simulink model "DatcomNew"  (R2017a)
settings: Solver=VariableStepAuto  StartTime=0.0  StopTime=10.0  RelTol=1e-3
undefined symbols (not defined in the file or in its folder): datcom, Newton, Raphson
libraries: aerolibutil x32, sharedutil x4, aerolibtransform2 x3, aerolibasang x3, aerolibadyn x1
(part 1 of 4)
settings Model: Creator=AHKh  LastModifiedBy=AHKh

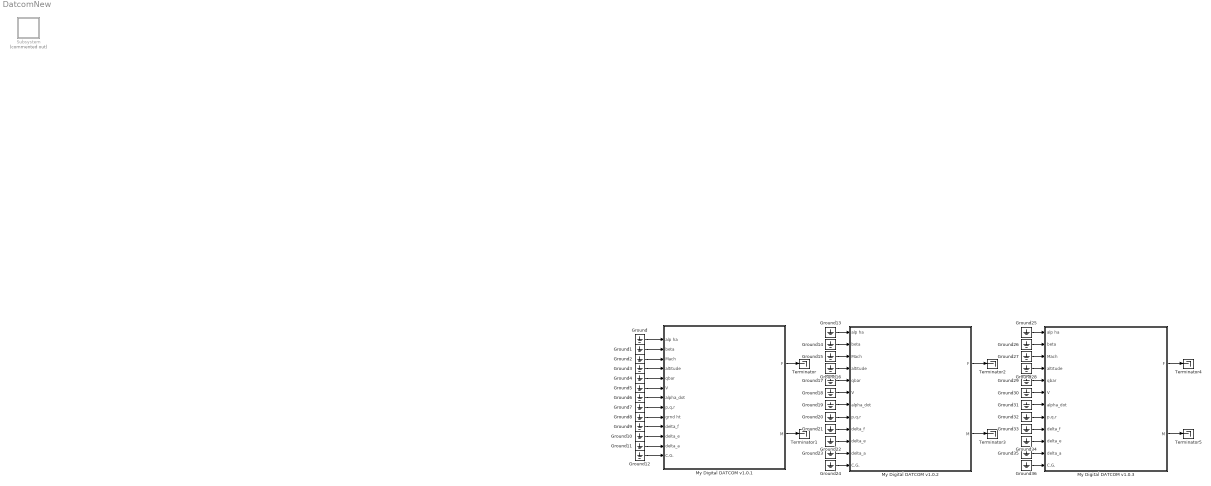
== system DatcomNew ==
  Ground{,1..36} (37 alike) : Ground
  My Digital DATCOM v1.0.1 : Subsystem  mask{datcom=datcom}
      mask prompts: datcom "Datcom Structure"
      mask Display:
      | port_label('input',1,'\alpha (rad)','texmode','on');
      | port_label('input',2,'\beta (rad)','texmode','on');
      | port_label('input',3,'Mach','texmode','on');
      | port_label('input',4,'h (m)','texmode','on');
      | port_label('input',5,'q_{bar}','texmode','on');
      | port_label('input',6,'V_{body} m/s','texmode','on');
      | port_label('input',7,'d\alpha/dt (rad/s)','texmode','on');
      | port_label('input',8,'\omega (rad/s)','texmode','on');
      | port_label('input',9,'h_{grnd} (m)','texmode','on');
      | port_label('input',10,'\delta_F (rad)','texmode','on');
      | port_label('input',11,'\delta_E (rad)','texmode','on');
      | port_label('input',12,'\delta_A (rad)','texmode','on');
      | port_label('input',13,'C.G. (m)','texmode','on');
      | port_label('output',1,'F_{body} (N)','texmode','on');
      | port_label('output',2,'M_{body} (N.m)','texmode','on');
  My Digital DATCOM v1.0.2 : Subsystem  mask{datcom=datcom}
      mask prompts: datcom "Datcom Structure"
      mask Display:
      | port_label('input',1,'\alpha (rad)','texmode','on');
      | port_label('input',2,'\beta (rad)','texmode','on');
      | port_label('input',3,'Mach','texmode','on');
      | port_label('input',4,'h (m)','texmode','on');
      | port_label('input',5,'q_{bar}','texmode','on');
      | port_label('input',6,'V_{body} m/s','texmode','on');
      | port_label('input',7,'d\alpha/dt (rad/s)','texmode','on');
      | port_label('input',8,'\omega (rad/s)','texmode','on');
      | port_label('input',9,'\delta_F (rad)','texmode','on');
      | port_label('input',10,'\delta_E (rad)','texmode','on');
      | port_label('input',11,'\delta_A (rad)','texmode','on');
      | port_label('input',12,'C.G. (m)','texmode','on');
      | port_label('output',1,'F_{body} (N)','texmode','on');
      | port_label('output',2,'M_{body} (N.m)','texmode','on');
  My Digital DATCOM v1.0.3 : Subsystem  mask{datcom=datcom}
      mask prompts: datcom "Datcom Structure"
      mask Display:
      | port_label('input',1,'\alpha (rad)','texmode','on');
      | port_label('input',2,'\beta (rad)','texmode','on');
      | port_label('input',3,'Mach','texmode','on');
      | port_label('input',4,'h (m)','texmode','on');
      | port_label('input',5,'q_{bar}','texmode','on');
      | port_label('input',6,'V_{body} m/s','texmode','on');
      | port_label('input',7,'d\alpha/dt (rad/s)','texmode','on');
      | port_label('input',8,'\omega (rad/s)','texmode','on');
      | port_label('input',9,'\delta_F (rad)','texmode','on');
      | port_label('input',10,'\delta_E (rad)','texmode','on');
      | port_label('input',11,'\delta_A (rad)','texmode','on');
      | port_label('input',12,'C.G. (m)','texmode','on');
      | port_label('output',1,'F_{body} (N)','texmode','on');
      | port_label('output',2,'M_{body} (N.m)','texmode','on');
  Subsystem : Subsystem  Commented=on
  Terminator{,1..5} (6 alike) : Terminator
  wires:
  My Digital DATCOM v1.0.1/2(M) -> Terminator1/1
  My Digital DATCOM v1.0.1/1(F) -> Terminator/1
  Ground4/1 -> My Digital DATCOM v1.0.1/5(qbar)
  Ground5/1 -> My Digital DATCOM v1.0.1/6(V)
  Ground/1 -> My Digital DATCOM v1.0.1/1(alp ha)
  Ground3/1 -> My Digital DATCOM v1.0.1/4(altitude)
  Ground7/1 -> My Digital DATCOM v1.0.1/8(p,q,r)
  Ground12/1 -> My Digital DATCOM v1.0.1/13(C.G.)
  Ground8/1 -> My Digital DATCOM v1.0.1/9(grnd ht)
  Ground6/1 -> My Digital DATCOM v1.0.1/7(alpha_dot)
  Ground1/1 -> My Digital DATCOM v1.0.1/2(beta)
  Ground2/1 -> My Digital DATCOM v1.0.1/3(Mach)
  Ground9/1 -> My Digital DATCOM v1.0.1/10(delta_f)
  Ground10/1 -> My Digital DATCOM v1.0.1/11(delta_e)
  Ground11/1 -> My Digital DATCOM v1.0.1/12(delta_a)
  My Digital DATCOM v1.0.2/1(F) -> Terminator2/1
  My Digital DATCOM v1.0.2/2(M) -> Terminator3/1
  Ground13/1 -> My Digital DATCOM v1.0.2/1(alp ha)
  Ground16/1 -> My Digital DATCOM v1.0.2/4(altitude)
  Ground19/1 -> My Digital DATCOM v1.0.2/7(alpha_dot)
  Ground18/1 -> My Digital DATCOM v1.0.2/6(V)
  Ground14/1 -> My Digital DATCOM v1.0.2/2(beta)
  Ground15/1 -> My Digital DATCOM v1.0.2/3(Mach)
  Ground17/1 -> My Digital DATCOM v1.0.2/5(qbar)
  Ground20/1 -> My Digital DATCOM v1.0.2/8(p,q,r)
  Ground22/1 -> My Digital DATCOM v1.0.2/10(delta_e)
  Ground21/1 -> My Digital DATCOM v1.0.2/9(delta_f)
  Ground24/1 -> My Digital DATCOM v1.0.2/12(C.G.)
  Ground23/1 -> My Digital DATCOM v1.0.2/11(delta_a)
  Ground27/1 -> My Digital DATCOM v1.0.3/3(Mach)
  My Digital DATCOM v1.0.3/2(M) -> Terminator5/1
  My Digital DATCOM v1.0.3/1(F) -> Terminator4/1
  Ground32/1 -> My Digital DATCOM v1.0.3/8(p,q,r)
  Ground26/1 -> My Digital DATCOM v1.0.3/2(beta)
  Ground33/1 -> My Digital DATCOM v1.0.3/9(delta_f)
  Ground29/1 -> My Digital DATCOM v1.0.3/5(qbar)
  Ground35/1 -> My Digital DATCOM v1.0.3/11(delta_a)
  Ground25/1 -> My Digital DATCOM v1.0.3/1(alp ha)
  Ground36/1 -> My Digital DATCOM v1.0.3/12(C.G.)
  Ground31/1 -> My Digital DATCOM v1.0.3/7(alpha_dot)
  Ground30/1 -> My Digital DATCOM v1.0.3/6(V)
  Ground28/1 -> My Digital DATCOM v1.0.3/4(altitude)
  Ground34/1 -> My Digital DATCOM v1.0.3/10(delta_e)

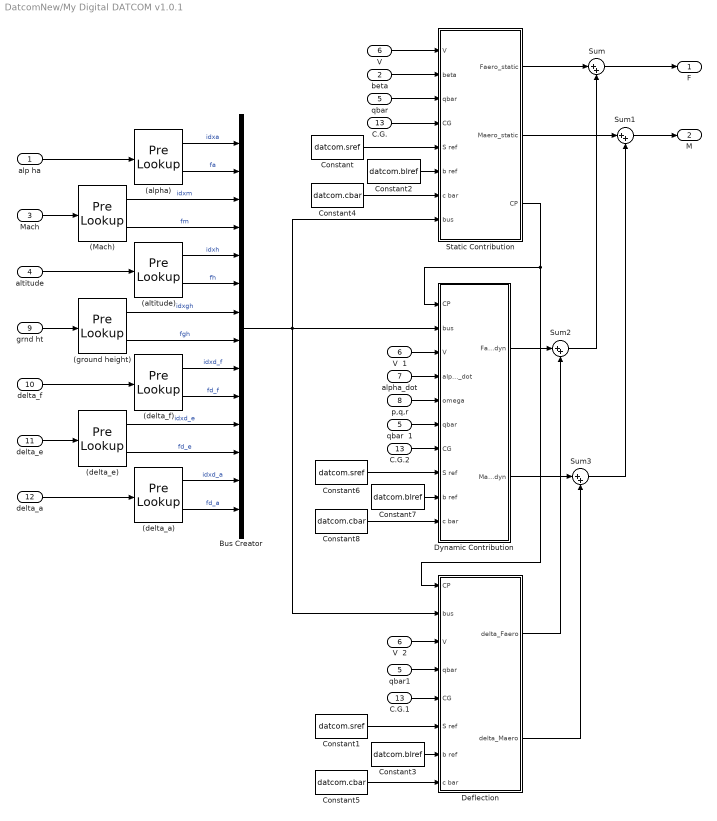
== system DatcomNew/My Digital DATCOM v1.0.1 ==
  alp ha : Inport  Unit=rad
  beta : Inport  Port=2  Unit=rad
  Mach : Inport  Port=3  Unit=1
  altitude : Inport  Port=4  Unit=m
  qbar : Inport  Port=5  Unit=Pa
  V : Inport  Port=6  Unit=m/s
  alpha_dot : Inport  Port=7  Unit=rad/s
  p,q,r : Inport  Port=8  Unit=rad/s
  grnd ht : Inport  Port=9  Unit=m
  delta_f : Inport  Port=10  Unit=rad
  delta_e : Inport  Port=11  Unit=rad
  delta_a : Inport  Port=12  Unit=rad
  C.G. : Inport  Port=13  Unit=m
  (Mach) : PreLookup  BreakpointsData=datcom.mach  BeginIndexSearchUsingPreviousIndexResult=on  IndexDataTypeStr=int32  FractionDataTypeStr=double
  (alpha) : PreLookup  BreakpointsData=datcom.alpha  BeginIndexSearchUsingPreviousIndexResult=on  IndexDataTypeStr=int32  FractionDataTypeStr=double
  (altitude) : PreLookup  BreakpointsData=datcom.alt  BeginIndexSearchUsingPreviousIndexResult=on  IndexDataTypeStr=int32  FractionDataTypeStr=double
  (delta_a) : PreLookup  BreakpointsData=datcom.deltal-datcom.deltar  BeginIndexSearchUsingPreviousIndexResult=on  IndexDataTypeStr=int32  FractionDataTypeStr=double
  (delta_e) : PreLookup  BreakpointsData=datcom.delta  BeginIndexSearchUsingPreviousIndexResult=on  IndexDataTypeStr=int32  FractionDataTypeStr=double
  (delta_f) : PreLookup  BreakpointsData=datcom.delta  BeginIndexSearchUsingPreviousIndexResult=on  IndexDataTypeStr=int32  FractionDataTypeStr=double
  (ground height) : PreLookup  BreakpointsData=[0:2]  BeginIndexSearchUsingPreviousIndexResult=on  IndexDataTypeStr=int32  FractionDataTypeStr=double
  Bus Creator : BusCreator  Inputs=14
  C.G.1 : InportShadow  Port=13  Unit=m
  C.G.2 : InportShadow  Port=13  Unit=m
  Constant : Constant  Value=datcom.sref
  Constant1 : Constant  Value=datcom.sref
  Constant2 : Constant  Value=datcom.blref
  Constant3 : Constant  Value=datcom.blref
  Constant4 : Constant  Value=datcom.cbar
  Constant5 : Constant  Value=datcom.cbar
  Constant6 : Constant  Value=datcom.sref
  Constant7 : Constant  Value=datcom.blref
  Constant8 : Constant  Value=datcom.cbar
  Deflection : Subsystem
  Dynamic Contribution : Subsystem
  Static Contribution : Subsystem
  Sum{,1..3} (4 alike) : Sum  Inputs=|++
  V  1 : InportShadow  Port=6  Unit=m/s
  V  2 : InportShadow  Port=6  Unit=m/s
  qbar  1 : InportShadow  Port=5  Unit=Pa
  qbar1 : InportShadow  Port=5  Unit=Pa
  F : Outport  Unit=N
  M : Outport  Port=2  Unit=N*m
  wires:
  Bus Creator/1 -> Static Contribution/8(bus), Dynamic Contribution/2(bus), Deflection/2(bus)
  delta_f/1 -> (delta_f)/1
  (alpha)/1 -> Bus Creator/1  "idxa"
  (Mach)/1 -> Bus Creator/3  "idxm"
  Mach/1 -> (Mach)/1
  Static Contribution/3("CP ") -> Dynamic Contribution/1(CP), Deflection/1(CP)
  Static Contribution/1(Faero_static) -> Sum/1
  Dynamic Contribution/1(Faero_dyn) -> Sum2/1
  Static Contribution/2(Maero_static) -> Sum1/1
  Dynamic Contribution/2(Maero_dyn) -> Sum3/1
  Sum/1 -> F/1
  Sum1/1 -> M/1
  alpha_dot/1 -> Dynamic Contribution/4(alpha_dot)
  p,q,r/1 -> Dynamic Contribution/5(omega)
  qbar  1/1 -> Dynamic Contribution/6(qbar)
  altitude/1 -> (altitude)/1
  grnd ht/1 -> (ground height)/1
  (delta_f)/1 -> Bus Creator/9  "idxd_f"
  (delta_f)/2 -> Bus Creator/10  "fd_f"
  (ground height)/1 -> Bus Creator/7  "idxgh"
  (ground height)/2 -> Bus Creator/8  "fgh"
  (altitude)/1 -> Bus Creator/5  "idxh"
  (altitude)/2 -> Bus Creator/6  "fh"
  (Mach)/2 -> Bus Creator/4  "fm"
  (alpha)/2 -> Bus Creator/2  "fa"
  alp ha/1 -> (alpha)/1
  beta/1 -> Static Contribution/2(beta)
  qbar/1 -> Static Contribution/3(qbar)
  V  1/1 -> Dynamic Contribution/3(V)
  V/1 -> Static Contribution/1("V ")
  delta_e/1 -> (delta_e)/1
  (delta_e)/1 -> Bus Creator/11  "idxd_e"
  (delta_e)/2 -> Bus Creator/12  "fd_e"
  delta_a/1 -> (delta_a)/1
  (delta_a)/1 -> Bus Creator/13  "idxd_a"
  (delta_a)/2 -> Bus Creator/14  "fd_a"
  V  2/1 -> Deflection/3("V ")
  qbar1/1 -> Deflection/4(qbar)
  Sum2/1 -> Sum/2
  Sum3/1 -> Sum1/2
  Deflection/1(delta_Faero) -> Sum2/2
  Deflection/2(delta_Maero) -> Sum3/2
  C.G./1 -> Static Contribution/4(CG)
  C.G.1/1 -> Deflection/5(CG)
  Constant/1 -> Static Contribution/5(S ref)
  Constant1/1 -> Deflection/6(S ref)
  Constant2/1 -> Static Contribution/6(b ref)
  Constant3/1 -> Deflection/7(b ref)
  Constant5/1 -> Deflection/8(c bar)
  Constant4/1 -> Static Contribution/7(c bar)
  C.G.2/1 -> Dynamic Contribution/7(CG)
  Constant7/1 -> Dynamic Contribution/9(b ref)
  Constant6/1 -> Dynamic Contribution/8(S ref)
  Constant8/1 -> Dynamic Contribution/10(c bar)

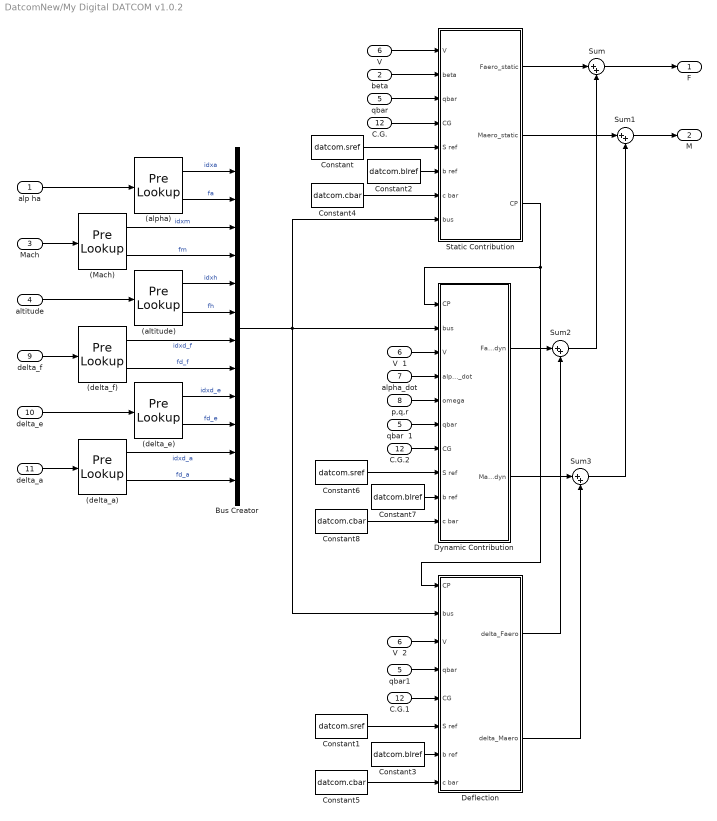
== system DatcomNew/My Digital DATCOM v1.0.2 ==
  alp ha : Inport  Unit=rad
  beta : Inport  Port=2  Unit=rad
  Mach : Inport  Port=3  Unit=1
  altitude : Inport  Port=4  Unit=m
  qbar : Inport  Port=5  Unit=Pa
  V : Inport  Port=6  Unit=m/s
  alpha_dot : Inport  Port=7  Unit=rad/s
  p,q,r : Inport  Port=8  Unit=rad/s
  delta_f : Inport  Port=9  Unit=rad
  delta_e : Inport  Port=10  Unit=rad
  delta_a : Inport  Port=11  Unit=rad
  C.G. : Inport  Port=12  Unit=m
  (Mach) : PreLookup  BreakpointsData=datcom.mach  BeginIndexSearchUsingPreviousIndexResult=on  IndexDataTypeStr=int32  FractionDataTypeStr=double
  (alpha) : PreLookup  BreakpointsData=datcom.alpha  BeginIndexSearchUsingPreviousIndexResult=on  IndexDataTypeStr=int32  FractionDataTypeStr=double
  (altitude) : PreLookup  BreakpointsData=datcom.alt  BeginIndexSearchUsingPreviousIndexResult=on  IndexDataTypeStr=int32  FractionDataTypeStr=double
  (delta_a) : PreLookup  BreakpointsData=datcom.deltal-datcom.deltar  BeginIndexSearchUsingPreviousIndexResult=on  IndexDataTypeStr=int32  FractionDataTypeStr=double
  (delta_e) : PreLookup  BreakpointsData=datcom.delta  BeginIndexSearchUsingPreviousIndexResult=on  IndexDataTypeStr=int32  FractionDataTypeStr=double
  (delta_f) : PreLookup  BreakpointsData=datcom.delta  BeginIndexSearchUsingPreviousIndexResult=on  IndexDataTypeStr=int32  FractionDataTypeStr=double
  Bus Creator : BusCreator  Inputs=12
  C.G.1 : InportShadow  Port=12  Unit=m
  C.G.2 : InportShadow  Port=12  Unit=m
  Constant : Constant  Value=datcom.sref
  Constant1 : Constant  Value=datcom.sref
  Constant2 : Constant  Value=datcom.blref
  Constant3 : Constant  Value=datcom.blref
  Constant4 : Constant  Value=datcom.cbar
  Constant5 : Constant  Value=datcom.cbar
  Constant6 : Constant  Value=datcom.sref
  Constant7 : Constant  Value=datcom.blref
  Constant8 : Constant  Value=datcom.cbar
  Deflection : Subsystem
  Dynamic Contribution : Subsystem
  Static Contribution : Subsystem
  Sum{,1..3} (4 alike) : Sum  Inputs=|++
  V  1 : InportShadow  Port=6  Unit=m/s
  V  2 : InportShadow  Port=6  Unit=m/s
  qbar  1 : InportShadow  Port=5  Unit=Pa
  qbar1 : InportShadow  Port=5  Unit=Pa
  F : Outport  Unit=N
  M : Outport  Port=2  Unit=N*m
  wires:
  Constant8/1 -> Dynamic Contribution/10(c bar)
  Constant6/1 -> Dynamic Contribution/8(S ref)
  Constant7/1 -> Dynamic Contribution/9(b ref)
  C.G.2/1 -> Dynamic Contribution/7(CG)
  Constant4/1 -> Static Contribution/7(c bar)
  Constant5/1 -> Deflection/8(c bar)
  Constant3/1 -> Deflection/7(b ref)
  Constant2/1 -> Static Contribution/6(b ref)
  Constant1/1 -> Deflection/6(S ref)
  Constant/1 -> Static Contribution/5(S ref)
  C.G.1/1 -> Deflection/5(CG)
  C.G./1 -> Static Contribution/4(CG)
  Deflection/2(delta_Maero) -> Sum3/2
  Deflection/1(delta_Faero) -> Sum2/2
  Sum3/1 -> Sum1/2
  Sum2/1 -> Sum/2
  qbar1/1 -> Deflection/4(qbar)
  V  2/1 -> Deflection/3("V ")
  (delta_a)/2 -> Bus Creator/12  "fd_a"
  (delta_a)/1 -> Bus Creator/11  "idxd_a"
  delta_a/1 -> (delta_a)/1
  (delta_e)/2 -> Bus Creator/10  "fd_e"
  (delta_e)/1 -> Bus Creator/9  "idxd_e"
  delta_e/1 -> (delta_e)/1
  V/1 -> Static Contribution/1("V ")
  V  1/1 -> Dynamic Contribution/3(V)
  qbar/1 -> Static Contribution/3(qbar)
  beta/1 -> Static Contribution/2(beta)
  alp ha/1 -> (alpha)/1
  (alpha)/2 -> Bus Creator/2  "fa"
  (Mach)/2 -> Bus Creator/4  "fm"
  (altitude)/2 -> Bus Creator/6  "fh"
  (altitude)/1 -> Bus Creator/5  "idxh"
  (delta_f)/2 -> Bus Creator/8  "fd_f"
  (delta_f)/1 -> Bus Creator/7  "idxd_f"
  altitude/1 -> (altitude)/1
  qbar  1/1 -> Dynamic Contribution/6(qbar)
  p,q,r/1 -> Dynamic Contribution/5(omega)
  alpha_dot/1 -> Dynamic Contribution/4(alpha_dot)
  Sum1/1 -> M/1
  Sum/1 -> F/1
  Dynamic Contribution/2(Maero_dyn) -> Sum3/1
  Static Contribution/2(Maero_static) -> Sum1/1
  Dynamic Contribution/1(Faero_dyn) -> Sum2/1
  Static Contribution/1(Faero_static) -> Sum/1
  Static Contribution/3("CP ") -> Deflection/1(CP), Dynamic Contribution/1(CP)
  Mach/1 -> (Mach)/1
  (Mach)/1 -> Bus Creator/3  "idxm"
  (alpha)/1 -> Bus Creator/1  "idxa"
  delta_f/1 -> (delta_f)/1
  Bus Creator/1 -> Deflection/2(bus), Dynamic Contribution/2(bus), Static Contribution/8(bus)

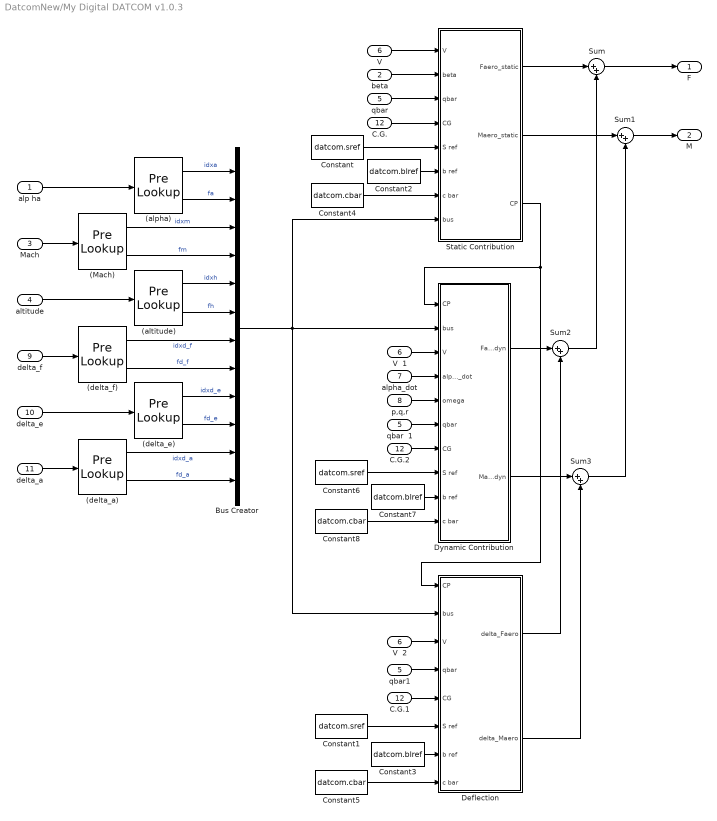
== system DatcomNew/My Digital DATCOM v1.0.3 ==
  alp ha : Inport  Unit=rad
  beta : Inport  Port=2  Unit=rad
  Mach : Inport  Port=3  Unit=1
  altitude : Inport  Port=4  Unit=m
  qbar : Inport  Port=5  Unit=Pa
  V : Inport  Port=6  Unit=m/s
  alpha_dot : Inport  Port=7  Unit=rad/s
  p,q,r : Inport  Port=8  Unit=rad/s
  delta_f : Inport  Port=9  Unit=rad
  delta_e : Inport  Port=10  Unit=rad
  delta_a : Inport  Port=11  Unit=rad
  C.G. : Inport  Port=12  Unit=m
  (Mach) : PreLookup  BreakpointsData=datcom.mach  BeginIndexSearchUsingPreviousIndexResult=on  IndexDataTypeStr=int32  FractionDataTypeStr=double
  (alpha) : PreLookup  BreakpointsData=datcom.alpha  BeginIndexSearchUsingPreviousIndexResult=on  IndexDataTypeStr=int32  FractionDataTypeStr=double
  (altitude) : PreLookup  BreakpointsData=datcom.alt  BeginIndexSearchUsingPreviousIndexResult=on  IndexDataTypeStr=int32  FractionDataTypeStr=double
  (delta_a) : PreLookup  BreakpointsData=datcom.deltal-datcom.deltar  BeginIndexSearchUsingPreviousIndexResult=on  IndexDataTypeStr=int32  FractionDataTypeStr=double
  (delta_e) : PreLookup  BreakpointsData=datcom.delta  BeginIndexSearchUsingPreviousIndexResult=on  IndexDataTypeStr=int32  FractionDataTypeStr=double
  (delta_f) : PreLookup  BreakpointsData=datcom.delta  BeginIndexSearchUsingPreviousIndexResult=on  IndexDataTypeStr=int32  FractionDataTypeStr=double
  Bus Creator : BusCreator  Inputs=12
  C.G.1 : InportShadow  Port=12  Unit=m
  C.G.2 : InportShadow  Port=12  Unit=m
  Constant : Constant  Value=datcom.sref
  Constant1 : Constant  Value=datcom.sref
  Constant2 : Constant  Value=datcom.blref
  Constant3 : Constant  Value=datcom.blref
  Constant4 : Constant  Value=datcom.cbar
  Constant5 : Constant  Value=datcom.cbar
  Constant6 : Constant  Value=datcom.sref
  Constant7 : Constant  Value=datcom.blref
  Constant8 : Constant  Value=datcom.cbar
  Deflection : Subsystem
  Dynamic Contribution : Subsystem
  Static Contribution : Subsystem
  Sum{,1..3} (4 alike) : Sum  Inputs=|++
  V  1 : InportShadow  Port=6  Unit=m/s
  V  2 : InportShadow  Port=6  Unit=m/s
  qbar  1 : InportShadow  Port=5  Unit=Pa
  qbar1 : InportShadow  Port=5  Unit=Pa
  F : Outport  Unit=N
  M : Outport  Port=2  Unit=N*m
  wires:
  Constant8/1 -> Dynamic Contribution/10(c bar)
  Constant6/1 -> Dynamic Contribution/8(S ref)
  Constant7/1 -> Dynamic Contribution/9(b ref)
  C.G.2/1 -> Dynamic Contribution/7(CG)
  Constant4/1 -> Static Contribution/7(c bar)
  Constant5/1 -> Deflection/8(c bar)
  Constant3/1 -> Deflection/7(b ref)
  Constant2/1 -> Static Contribution/6(b ref)
  Constant1/1 -> Deflection/6(S ref)
  Constant/1 -> Static Contribution/5(S ref)
  C.G.1/1 -> Deflection/5(CG)
  C.G./1 -> Static Contribution/4(CG)
  Deflection/2(delta_Maero) -> Sum3/2
  Deflection/1(delta_Faero) -> Sum2/2
  Sum3/1 -> Sum1/2
  Sum2/1 -> Sum/2
  qbar1/1 -> Deflection/4(qbar)
  V  2/1 -> Deflection/3("V ")
  (delta_a)/2 -> Bus Creator/12  "fd_a"
  (delta_a)/1 -> Bus Creator/11  "idxd_a"
  delta_a/1 -> (delta_a)/1
  (delta_e)/2 -> Bus Creator/10  "fd_e"
  (delta_e)/1 -> Bus Creator/9  "idxd_e"
  delta_e/1 -> (delta_e)/1
  V/1 -> Static Contribution/1("V ")
  V  1/1 -> Dynamic Contribution/3(V)
  qbar/1 -> Static Contribution/3(qbar)
  beta/1 -> Static Contribution/2(beta)
  alp ha/1 -> (alpha)/1
  (alpha)/2 -> Bus Creator/2  "fa"
  (Mach)/2 -> Bus Creator/4  "fm"
  (altitude)/2 -> Bus Creator/6  "fh"
  (altitude)/1 -> Bus Creator/5  "idxh"
  (delta_f)/2 -> Bus Creator/8  "fd_f"
  (delta_f)/1 -> Bus Creator/7  "idxd_f"
  altitude/1 -> (altitude)/1
  qbar  1/1 -> Dynamic Contribution/6(qbar)
  p,q,r/1 -> Dynamic Contribution/5(omega)
  alpha_dot/1 -> Dynamic Contribution/4(alpha_dot)
  Sum1/1 -> M/1
  Sum/1 -> F/1
  Dynamic Contribution/2(Maero_dyn) -> Sum3/1
  Static Contribution/2(Maero_static) -> Sum1/1
  Dynamic Contribution/1(Faero_dyn) -> Sum2/1
  Static Contribution/1(Faero_static) -> Sum/1
  Static Contribution/3("CP ") -> Deflection/1(CP), Dynamic Contribution/1(CP)
  Mach/1 -> (Mach)/1
  (Mach)/1 -> Bus Creator/3  "idxm"
  (alpha)/1 -> Bus Creator/1  "idxa"
  delta_f/1 -> (delta_f)/1
  Bus Creator/1 -> Deflection/2(bus), Dynamic Contribution/2(bus), Static Contribution/8(bus)

== system DatcomNew/Subsystem ==
  Digital DATCOM Forces and Moments : aerolibadyn/Digital DATCOM Forces and Moments  Commented=on  units=Metric (MKS)  dcase=datcom  fmode=Body  buildno=0  imethod=None - flat  emethod=None - clip  rmethod=Clip to Range  action=None
      settings: SourceProductName=Aerospace Blockset  SourceProductBaseCode=AE
  Unit System Configuration : UnitConfiguration  Commented=on  UnitSystemsStr=English,SI,SI (extended)  AllowAllUnitSystems=off

== system DatcomNew/My Digital DATCOM v1.0.1/Deflection ==
  CP : Inport
  bus : Inport  Port=2
  "V " : Inport  Port=3
  qbar : Inport  Port=4
  CG : Inport  Port=5
  S ref : Inport  Port=6  Unit=m^2
  b ref : Inport  Port=7  Unit=m  PortDimensions=1
  c bar : Inport  Port=8  Unit=m  PortDimensions=1
  Aerodynamic Forces and Moments : Subsystem
  Delta Coefficients : Subsystem
  delta_Faero : Outport
  delta_Maero : Outport  Port=2
  wires:
  bus/1 -> Delta Coefficients/1(bus)
  Delta Coefficients/1(delCoeff) -> Aerodynamic Forces and Moments/1(Coefficients)
  CP/1 -> Aerodynamic Forces and Moments/4(CP)
  "V "/1 -> Aerodynamic Forces and Moments/5(Vb)
  CG/1 -> Aerodynamic Forces and Moments/3(CG)
  c bar/1 -> Aerodynamic Forces and Moments/8(cbar)
  qbar/1 -> Aerodynamic Forces and Moments/2(qbar)
  b ref/1 -> Aerodynamic Forces and Moments/7(b ref)
  S ref/1 -> Aerodynamic Forces and Moments/6(S ref)
  Aerodynamic Forces and Moments/2(Moments) -> delta_Maero/1
  Aerodynamic Forces and Moments/1(Forces) -> delta_Faero/1

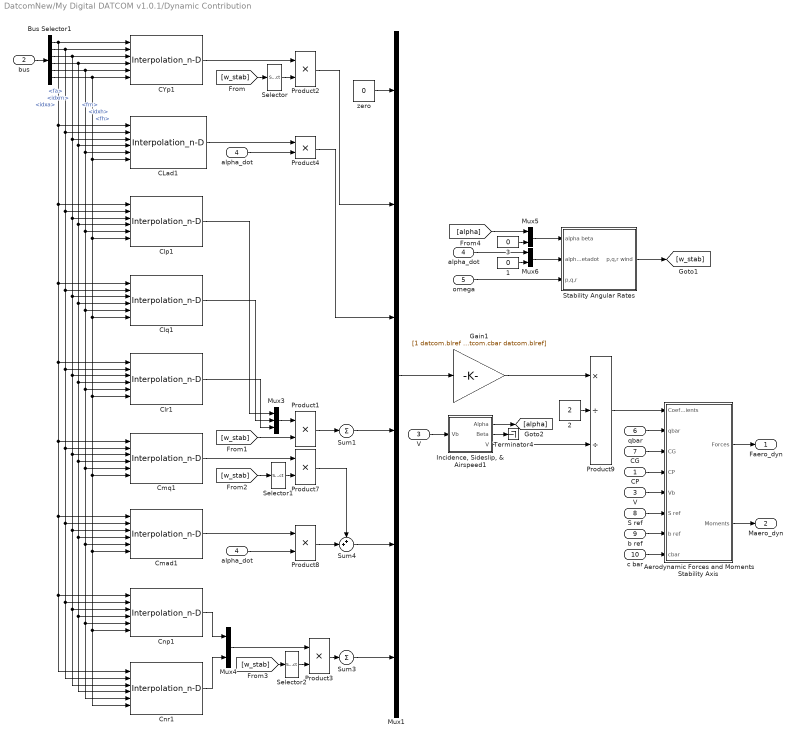
== system DatcomNew/My Digital DATCOM v1.0.1/Dynamic Contribution ==
  CP : Inport
  bus : Inport  Port=2
  V : Inport  Port=3
  alpha_dot : Inport  Port=4  Unit=rad/s
  omega : Inport  Port=5  Unit=rad/s
  qbar : Inport  Port=6
  CG : Inport  Port=7
  S ref : Inport  Port=8  Unit=m^2
  b ref : Inport  Port=9  Unit=m  PortDimensions=1
  c bar : Inport  Port=10  Unit=m  PortDimensions=1
  " V " : InportShadow  Port=3
  " alpha_dot " : InportShadow  Port=4  Unit=rad/s
  1 : Constant  Value=0
  2 : Constant  Value=2
  3 : Constant  Value=0
  Aerodynamic Forces and Moments Stability Axis : Subsystem
  Bus Selector1 : BusSelector  OutputSignals=idxa,fa,idxm,fm,idxh,fh
  CLad1 : Interpolation_n-D  NumberOfTableDimensions=3  Table="permute(datcom.clad,[1  2  3])"  OutDataTypeStr=double
      settings: InputPortMap=u0,u1,u2,u3,u4,u5
  CYp1 : Interpolation_n-D  NumberOfTableDimensions=3  Table="permute(datcom.cyp,[1  2  3])"  OutDataTypeStr=double
      settings: InputPortMap=u0,u1,u2,u3,u4,u5
  Clp1 : Interpolation_n-D  NumberOfTableDimensions=3  Table="permute(datcom.clp,[1  2  3])"  OutDataTypeStr=double
      settings: InputPortMap=u0,u1,u2,u3,u4,u5
  Clq1 : Interpolation_n-D  NumberOfTableDimensions=3  Table="permute(datcom.clq,[1  2  3])"  OutDataTypeStr=double
      settings: InputPortMap=u0,u1,u2,u3,u4,u5
  Clr1 : Interpolation_n-D  NumberOfTableDimensions=3  Table="permute(datcom.clr,[1  2  3])"  OutDataTypeStr=double
      settings: InputPortMap=u0,u1,u2,u3,u4,u5
  Cmad1 : Interpolation_n-D  NumberOfTableDimensions=3  Table="permute(datcom.cmad,[1  2  3])"  OutDataTypeStr=double
      settings: InputPortMap=u0,u1,u2,u3,u4,u5
  Cmq1 : Interpolation_n-D  NumberOfTableDimensions=3  Table="permute(datcom.cmq,[1  2  3])"  OutDataTypeStr=double
      settings: InputPortMap=u0,u1,u2,u3,u4,u5
  Cnp1 : Interpolation_n-D  NumberOfTableDimensions=3  Table="permute(datcom.cnp,[1  2  3])"  OutDataTypeStr=double
      settings: InputPortMap=u0,u1,u2,u3,u4,u5
  Cnr1 : Interpolation_n-D  NumberOfTableDimensions=3  Table="permute(datcom.cnr,[1  2  3])"  OutDataTypeStr=double
      settings: InputPortMap=u0,u1,u2,u3,u4,u5
  Gain1 : Gain  Gain=[1 datcom.blref datcom.cbar datcom.blref datcom.cbar datcom.blref]
  "Incidence, Sideslip, & Airspeed1" : Subsystem
      mask Display:
      | port_label('input',1,'V_b','texmode','on');
      | port_label('output',1,'\alpha','texmode','on');
      | port_label('output',2,'\beta','texmode','on');
      | port_label('output',3,'V','texmode','on');
  Mux1 : Mux  Inputs=6
  Mux3 : Mux  Inputs=3
  Mux4 : Mux  Inputs=2
  Mux5 : Mux  Inputs=2
  Mux6 : Mux  Inputs=2
  Product{1..4,7..8} (6 alike) : Product  RndMeth=Zero
  Product9 : Product  Inputs=*//  RndMeth=Zero
  Selector : Selector  InputPortWidth=3  IndexOptions=Index vector (dialog)  Indices=1  OutputSizes=1
  Selector1 : Selector  InputPortWidth=3  IndexOptions=Index vector (dialog)  Indices=2  OutputSizes=1
  Selector2 : Selector  InputPortWidth=3  IndexOptions=Index vector (dialog)  Indices=[1 3]  OutputSizes=1
  Stability Angular Rates : Subsystem
      mask Display:
      | port_label('input',1,'\alpha \beta','texmode','on');
      | port_label('input',2,'d\alpha/dt d\beta/dt','texmode','on');
      | port_label('input',3,'\omega','texmode','on');
      | port_label('output',1,'\omega_w','texmode','on');
  Sum1 : Sum  Inputs=+
  Sum3 : Sum  Inputs=+
  Sum4 : Sum  Inputs=++|
  Terminator4 : Terminator
  "alpha_dot " : InportShadow  Port=4  Unit=rad/s
  zero : Constant  Value=0
  Faero_dyn : Outport
  Maero_dyn : Outport  Port=2
  wires:
  CP/1 -> Aerodynamic Forces and Moments Stability Axis/4(CP)
  CG/1 -> Aerodynamic Forces and Moments Stability Axis/3(CG)
  1/1 -> Mux6/2
  Mux6/1 -> Stability Angular Rates/2(alphadot betadot)
  Mux5/1 -> Stability Angular Rates/1(alpha beta)
  [alpha] -> Mux5/1
  3/1 -> Mux5/2
  " V "/1 -> Aerodynamic Forces and Moments Stability Axis/5(Vb)
  Aerodynamic Forces and Moments Stability Axis/2(Moments) -> Maero_dyn/1
  qbar/1 -> Aerodynamic Forces and Moments Stability Axis/2(qbar)
  Aerodynamic Forces and Moments Stability Axis/1(Forces) -> Faero_dyn/1
  "Incidence, Sideslip, & Airspeed1"/1(Alpha) -> [alpha]
  "Incidence, Sideslip, & Airspeed1"/2(Beta) -> Terminator4/1
  "Incidence, Sideslip, & Airspeed1"/3(V) -> Product9/3
  zero/1 -> Mux1/1
  Product4/1 -> Mux1/3
  Sum4/1 -> Mux1/5
  V/1 -> "Incidence, Sideslip, & Airspeed1"/1(Vb)
  2/1 -> Product9/2
  Product9/1 -> Aerodynamic Forces and Moments Stability Axis/1(Coefficients)
  Gain1/1 -> Product9/1
  Product3/1 -> Sum3/1
  Sum3/1 -> Mux1/6
  Selector2/1 -> Product3/2
  Mux4/1 -> Product3/1
  [w_stab] -> Selector2/1
  Cnr1/1 -> Mux4/2
  alpha_dot/1 -> Product8/2
  Product8/1 -> Sum4/2
  Cmad1/1 -> Product8/1
  Product7/1 -> Sum4/1
  Selector1/1 -> Product7/2
  [w_stab] -> Selector1/1
  Product1/1 -> Sum1/1
  [w_stab] -> Product1/2
  Mux3/1 -> Product1/1
  Clp1/1 -> Mux3/1
  Clr1/1 -> Mux3/3
  [w_stab] -> Selector/1
  "alpha_dot "/1 -> Product4/2
  CYp1/1 -> Product2/1
  Selector/1 -> Product2/2
  Clq1/1 -> Mux3/2
  Product2/1 -> Mux1/2
  Sum1/1 -> Mux1/4
  Cmq1/1 -> Product7/1
  Cnp1/1 -> Mux4/1
  Mux1/1 -> Gain1/1
  Stability Angular Rates/1(p,q,r wind) -> [w_stab]
  omega/1 -> Stability Angular Rates/3(p,q,r)
  " alpha_dot "/1 -> Mux6/1
  bus/1 -> Bus Selector1/1
  Bus Selector1/1 -> CYp1/1, CLad1/1, Cnr1/1, Cnp1/1, Cmad1/1, Cmq1/1, Clr1/1, Clq1/1, Clp1/1  "<idxa>"
  Bus Selector1/2 -> CYp1/2, CLad1/2, Cnr1/2, Cnp1/2, Cmad1/2, Cmq1/2, Clr1/2, Clq1/2, Clp1/2  "<fa>"
  Bus Selector1/3 -> CYp1/3, CLad1/3, Cnr1/3, Cnp1/3, Cmad1/3, Cmq1/3, Clr1/3, Clq1/3, Clp1/3  "<idxm>"
  Bus Selector1/4 -> CYp1/4, CLad1/4, Cnr1/4, Cnp1/4, Cmad1/4, Cmq1/4, Clr1/4, Clq1/4, Clp1/4  "<fm>"
  Bus Selector1/5 -> CYp1/5, CLad1/5, Cnr1/5, Cnp1/5, Cmad1/5, Cmq1/5, Clr1/5, Clq1/5, Clp1/5  "<idxh>"
  Bus Selector1/6 -> CYp1/6, CLad1/6, Cnr1/6, Cnp1/6, Cmad1/6, Cmq1/6, Clr1/6, Clq1/6, Clp1/6  "<fh>"
  CLad1/1 -> Product4/1
  S ref/1 -> Aerodynamic Forces and Moments Stability Axis/6(S ref)
  b ref/1 -> Aerodynamic Forces and Moments Stability Axis/7(b ref)
  c bar/1 -> Aerodynamic Forces and Moments Stability Axis/8(cbar)

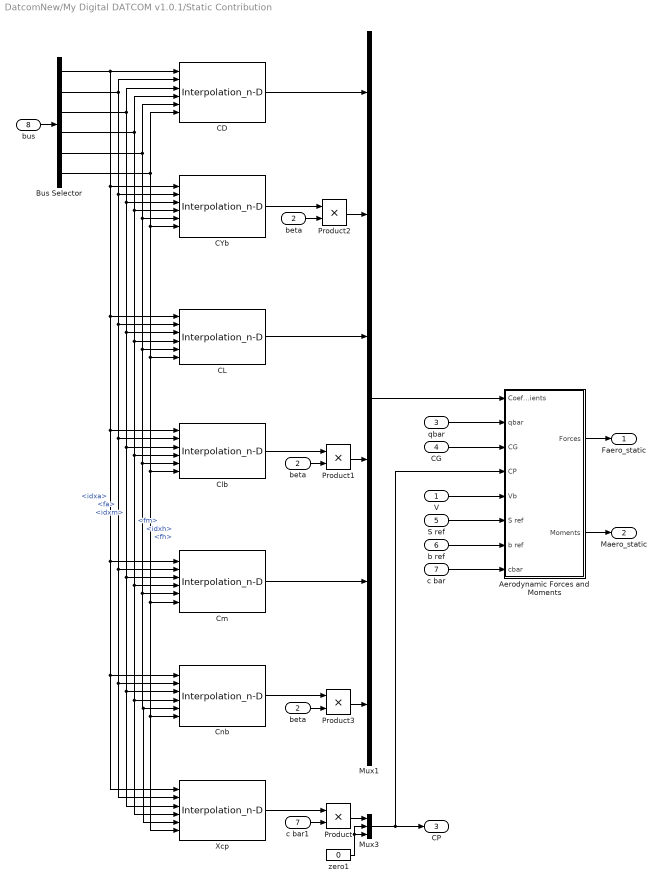
== system DatcomNew/My Digital DATCOM v1.0.1/Static Contribution ==
  "V " : Inport
  beta : Inport  Port=2
  qbar : Inport  Port=3
  CG : Inport  Port=4
  S ref : Inport  Port=5  Unit=m^2
  b ref : Inport  Port=6  Unit=m  PortDimensions=1
  c bar : Inport  Port=7  Unit=m  PortDimensions=1
  bus : Inport  Port=8
  " beta " : InportShadow  Port=2
  Aerodynamic Forces and Moments : Subsystem
  Bus Selector : BusSelector  OutputSignals=idxa,fa,idxm,fm,idxh,fh
  CD : Interpolation_n-D  NumberOfTableDimensions=3  Table=permute(datcom.cd,[1 2 3])  InterpMethod=Flat  ExtrapMethod=Clip  OutDataTypeStr=double
      settings: InputPortMap=u0,u1,u2,u3,u4,u5
  CL : Interpolation_n-D  NumberOfTableDimensions=3  Table=permute(datcom.cl,[1 2 3])  InterpMethod=Flat  ExtrapMethod=Clip  OutDataTypeStr=double
      settings: InputPortMap=u0,u1,u2,u3,u4,u5
  CYb : Interpolation_n-D  NumberOfTableDimensions=3  Table=permute(datcom.cyb,[1 2 3])  InterpMethod=Flat  ExtrapMethod=Clip  OutDataTypeStr=double
      settings: InputPortMap=u0,u1,u2,u3,u4,u5
  Clb : Interpolation_n-D  NumberOfTableDimensions=3  Table=permute(datcom.clb,[1 2 3])  InterpMethod=Flat  ExtrapMethod=Clip  OutDataTypeStr=double
      settings: InputPortMap=u0,u1,u2,u3,u4,u5
  Cm : Interpolation_n-D  NumberOfTableDimensions=3  Table=permute(datcom.cm,[1 2 3])  InterpMethod=Flat  ExtrapMethod=Clip  OutDataTypeStr=double
      settings: InputPortMap=u0,u1,u2,u3,u4,u5
  Cnb : Interpolation_n-D  NumberOfTableDimensions=3  Table=permute(datcom.cnb,[1 2 3])  InterpMethod=Flat  ExtrapMethod=Clip  OutDataTypeStr=double
      settings: InputPortMap=u0,u1,u2,u3,u4,u5
  Mux1 : Mux  Inputs=6
  Mux3 : Mux  Inputs=3
  Product : Product
  Product1 : Product  RndMeth=Zero
  Product2 : Product  RndMeth=Zero
  Product3 : Product  RndMeth=Zero
  Xcp : Interpolation_n-D  NumberOfTableDimensions=3  Table="permute(datcom.xcp,[1  2  3])"  OutDataTypeStr=double
      settings: InputPortMap=u0,u1,u2,u3,u4,u5
  "beta " : InportShadow  Port=2
  c bar1 : InportShadow  Port=7  Unit=m  PortDimensions=1
  zero1 : Constant  Value=0
  Faero_static : Outport
  Maero_static : Outport  Port=2
  "CP " : Outport  Port=3
  wires:
  "V "/1 -> Aerodynamic Forces and Moments/5(Vb)
  Aerodynamic Forces and Moments/2(Moments) -> Maero_static/1
  qbar/1 -> Aerodynamic Forces and Moments/2(qbar)
  Aerodynamic Forces and Moments/1(Forces) -> Faero_static/1
  Mux1/1 -> Aerodynamic Forces and Moments/1(Coefficients)
  Product3/1 -> Mux1/6
  " beta "/1 -> Product3/2
  Cnb/1 -> Product3/1
  Cm/1 -> Mux1/5
  Product1/1 -> Mux1/4
  Product2/1 -> Mux1/2
  "beta "/1 -> Product1/2
  Clb/1 -> Product1/1
  beta/1 -> Product2/2
  CYb/1 -> Product2/1
  CL/1 -> Mux1/3
  CD/1 -> Mux1/1
  Bus Selector/6 -> CD/6, CYb/6, CL/6, Clb/6, Cm/6, Xcp/6, Cnb/6  "<fh>"
  Bus Selector/5 -> CD/5, CYb/5, CL/5, Clb/5, Cm/5, Xcp/5, Cnb/5  "<idxh>"
  Bus Selector/4 -> CD/4, CYb/4, CL/4, Clb/4, Cm/4, Xcp/4, Cnb/4  "<fm>"
  Bus Selector/3 -> CD/3, CYb/3, CL/3, Clb/3, Cm/3, Xcp/3, Cnb/3  "<idxm>"
  Bus Selector/2 -> CD/2, CYb/2, CL/2, Clb/2, Cm/2, Xcp/2, Cnb/2  "<fa>"
  Bus Selector/1 -> CL/1, Cm/1, Xcp/1, Cnb/1, Clb/1, CYb/1, CD/1  "<idxa>"
  bus/1 -> Bus Selector/1
  CG/1 -> Aerodynamic Forces and Moments/3(CG)
  Mux3/1 -> "CP "/1, Aerodynamic Forces and Moments/4(CP)
  S ref/1 -> Aerodynamic Forces and Moments/6(S ref)
  b ref/1 -> Aerodynamic Forces and Moments/7(b ref)
  c bar/1 -> Aerodynamic Forces and Moments/8(cbar)
  Xcp/1 -> Product/1
  zero1/1 -> Mux3/2, Mux3/3
  Product/1 -> Mux3/1
  c bar1/1 -> Product/2

== system DatcomNew/My Digital DATCOM v1.0.2/Deflection ==
  CP : Inport
  bus : Inport  Port=2
  "V " : Inport  Port=3
  qbar : Inport  Port=4
  CG : Inport  Port=5
  S ref : Inport  Port=6  Unit=m^2
  b ref : Inport  Port=7  Unit=m  PortDimensions=1
  c bar : Inport  Port=8  Unit=m  PortDimensions=1
  Aerodynamic Forces and Moments : Subsystem
  Delta Coefficients : Subsystem
  delta_Faero : Outport
  delta_Maero : Outport  Port=2
  wires:
  Aerodynamic Forces and Moments/1(Forces) -> delta_Faero/1
  Aerodynamic Forces and Moments/2(Moments) -> delta_Maero/1
  S ref/1 -> Aerodynamic Forces and Moments/6(S ref)
  b ref/1 -> Aerodynamic Forces and Moments/7(b ref)
  qbar/1 -> Aerodynamic Forces and Moments/2(qbar)
  c bar/1 -> Aerodynamic Forces and Moments/8(cbar)
  CG/1 -> Aerodynamic Forces and Moments/3(CG)
  "V "/1 -> Aerodynamic Forces and Moments/5(Vb)
  CP/1 -> Aerodynamic Forces and Moments/4(CP)
  Delta Coefficients/1(delCoeff) -> Aerodynamic Forces and Moments/1(Coefficients)
  bus/1 -> Delta Coefficients/1(bus)

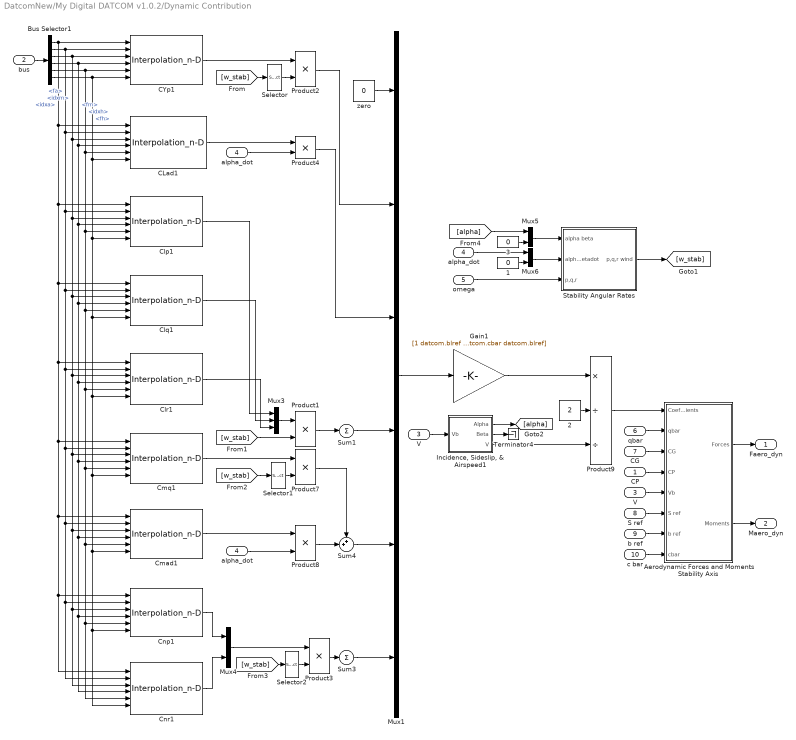
== system DatcomNew/My Digital DATCOM v1.0.2/Dynamic Contribution ==
  CP : Inport
  bus : Inport  Port=2
  V : Inport  Port=3
  alpha_dot : Inport  Port=4  Unit=rad/s
  omega : Inport  Port=5  Unit=rad/s
  qbar : Inport  Port=6
  CG : Inport  Port=7
  S ref : Inport  Port=8  Unit=m^2
  b ref : Inport  Port=9  Unit=m  PortDimensions=1
  c bar : Inport  Port=10  Unit=m  PortDimensions=1
  " V " : InportShadow  Port=3
  " alpha_dot " : InportShadow  Port=4  Unit=rad/s
  1 : Constant  Value=0
  2 : Constant  Value=2
  3 : Constant  Value=0
  Aerodynamic Forces and Moments Stability Axis : Subsystem
  Bus Selector1 : BusSelector  OutputSignals=idxa,fa,idxm,fm,idxh,fh
  CLad1 : Interpolation_n-D  NumberOfTableDimensions=3  Table="permute(datcom.clad,[1  2  3])"  OutDataTypeStr=double
      settings: InputPortMap=u0,u1,u2,u3,u4,u5
  CYp1 : Interpolation_n-D  NumberOfTableDimensions=3  Table="permute(datcom.cyp,[1  2  3])"  OutDataTypeStr=double
      settings: InputPortMap=u0,u1,u2,u3,u4,u5
  Clp1 : Interpolation_n-D  NumberOfTableDimensions=3  Table="permute(datcom.clp,[1  2  3])"  OutDataTypeStr=double
      settings: InputPortMap=u0,u1,u2,u3,u4,u5
  Clq1 : Interpolation_n-D  NumberOfTableDimensions=3  Table="permute(datcom.clq,[1  2  3])"  OutDataTypeStr=double
      settings: InputPortMap=u0,u1,u2,u3,u4,u5
  Clr1 : Interpolation_n-D  NumberOfTableDimensions=3  Table="permute(datcom.clr,[1  2  3])"  OutDataTypeStr=double
      settings: InputPortMap=u0,u1,u2,u3,u4,u5
  Cmad1 : Interpolation_n-D  NumberOfTableDimensions=3  Table="permute(datcom.cmad,[1  2  3])"  OutDataTypeStr=double
      settings: InputPortMap=u0,u1,u2,u3,u4,u5
  Cmq1 : Interpolation_n-D  NumberOfTableDimensions=3  Table="permute(datcom.cmq,[1  2  3])"  OutDataTypeStr=double
      settings: InputPortMap=u0,u1,u2,u3,u4,u5
  Cnp1 : Interpolation_n-D  NumberOfTableDimensions=3  Table="permute(datcom.cnp,[1  2  3])"  OutDataTypeStr=double
      settings: InputPortMap=u0,u1,u2,u3,u4,u5
  Cnr1 : Interpolation_n-D  NumberOfTableDimensions=3  Table="permute(datcom.cnr,[1  2  3])"  OutDataTypeStr=double
      settings: InputPortMap=u0,u1,u2,u3,u4,u5
  Gain1 : Gain  Gain=[1 datcom.blref datcom.cbar datcom.blref datcom.cbar datcom.blref]
  "Incidence, Sideslip, & Airspeed1" : Subsystem
      mask Display:
      | port_label('input',1,'V_b','texmode','on');
      | port_label('output',1,'\alpha','texmode','on');
      | port_label('output',2,'\beta','texmode','on');
      | port_label('output',3,'V','texmode','on');
  Mux1 : Mux  Inputs=6
  Mux3 : Mux  Inputs=3
  Mux4 : Mux  Inputs=2
  Mux5 : Mux  Inputs=2
  Mux6 : Mux  Inputs=2
  Product{1..4,7..8} (6 alike) : Product  RndMeth=Zero
  Product9 : Product  Inputs=*//  RndMeth=Zero
  Selector : Selector  InputPortWidth=3  IndexOptions=Index vector (dialog)  Indices=1  OutputSizes=1
  Selector1 : Selector  InputPortWidth=3  IndexOptions=Index vector (dialog)  Indices=2  OutputSizes=1
  Selector2 : Selector  InputPortWidth=3  IndexOptions=Index vector (dialog)  Indices=[1 3]  OutputSizes=1
  Stability Angular Rates : Subsystem
      mask Display:
      | port_label('input',1,'\alpha \beta','texmode','on');
      | port_label('input',2,'d\alpha/dt d\beta/dt','texmode','on');
      | port_label('input',3,'\omega','texmode','on');
      | port_label('output',1,'\omega_w','texmode','on');
  Sum1 : Sum  Inputs=+
  Sum3 : Sum  Inputs=+
  Sum4 : Sum  Inputs=++|
  Terminator4 : Terminator
  "alpha_dot " : InportShadow  Port=4  Unit=rad/s
  zero : Constant  Value=0
  Faero_dyn : Outport
  Maero_dyn : Outport  Port=2
  wires:
  c bar/1 -> Aerodynamic Forces and Moments Stability Axis/8(cbar)
  b ref/1 -> Aerodynamic Forces and Moments Stability Axis/7(b ref)
  S ref/1 -> Aerodynamic Forces and Moments Stability Axis/6(S ref)
  CLad1/1 -> Product4/1
  Bus Selector1/6 -> Clp1/6, Clq1/6, Clr1/6, Cmq1/6, Cmad1/6, Cnp1/6, Cnr1/6, CLad1/6, CYp1/6  "<fh>"
  Bus Selector1/5 -> Clp1/5, Clq1/5, Clr1/5, Cmq1/5, Cmad1/5, Cnp1/5, Cnr1/5, CLad1/5, CYp1/5  "<idxh>"
  Bus Selector1/4 -> Clp1/4, Clq1/4, Clr1/4, Cmq1/4, Cmad1/4, Cnp1/4, Cnr1/4, CLad1/4, CYp1/4  "<fm>"
  Bus Selector1/3 -> Clp1/3, Clq1/3, Clr1/3, Cmq1/3, Cmad1/3, Cnp1/3, Cnr1/3, CLad1/3, CYp1/3  "<idxm>"
  Bus Selector1/2 -> Clp1/2, Clq1/2, Clr1/2, Cmq1/2, Cmad1/2, Cnp1/2, Cnr1/2, CLad1/2, CYp1/2  "<fa>"
  Bus Selector1/1 -> Clp1/1, Clq1/1, Clr1/1, Cmq1/1, Cmad1/1, Cnp1/1, Cnr1/1, CLad1/1, CYp1/1  "<idxa>"
  bus/1 -> Bus Selector1/1
  " alpha_dot "/1 -> Mux6/1
  omega/1 -> Stability Angular Rates/3(p,q,r)
  Stability Angular Rates/1(p,q,r wind) -> [w_stab]
  Mux1/1 -> Gain1/1
  Cnp1/1 -> Mux4/1
  Cmq1/1 -> Product7/1
  Sum1/1 -> Mux1/4
  Product2/1 -> Mux1/2
  Clq1/1 -> Mux3/2
  Selector/1 -> Product2/2
  CYp1/1 -> Product2/1
  "alpha_dot "/1 -> Product4/2
  [w_stab] -> Selector/1
  Clr1/1 -> Mux3/3
  Clp1/1 -> Mux3/1
  Mux3/1 -> Product1/1
  [w_stab] -> Product1/2
  Product1/1 -> Sum1/1
  [w_stab] -> Selector1/1
  Selector1/1 -> Product7/2
  Product7/1 -> Sum4/1
  Cmad1/1 -> Product8/1
  Product8/1 -> Sum4/2
  alpha_dot/1 -> Product8/2
  Cnr1/1 -> Mux4/2
  [w_stab] -> Selector2/1
  Mux4/1 -> Product3/1
  Selector2/1 -> Product3/2
  Sum3/1 -> Mux1/6
  Product3/1 -> Sum3/1
  Gain1/1 -> Product9/1
  Product9/1 -> Aerodynamic Forces and Moments Stability Axis/1(Coefficients)
  2/1 -> Product9/2
  V/1 -> "Incidence, Sideslip, & Airspeed1"/1(Vb)
  Sum4/1 -> Mux1/5
  Product4/1 -> Mux1/3
  zero/1 -> Mux1/1
  "Incidence, Sideslip, & Airspeed1"/3(V) -> Product9/3
  "Incidence, Sideslip, & Airspeed1"/2(Beta) -> Terminator4/1
  "Incidence, Sideslip, & Airspeed1"/1(Alpha) -> [alpha]
  Aerodynamic Forces and Moments Stability Axis/1(Forces) -> Faero_dyn/1
  qbar/1 -> Aerodynamic Forces and Moments Stability Axis/2(qbar)
  Aerodynamic Forces and Moments Stability Axis/2(Moments) -> Maero_dyn/1
  " V "/1 -> Aerodynamic Forces and Moments Stability Axis/5(Vb)
  3/1 -> Mux5/2
  [alpha] -> Mux5/1
  Mux5/1 -> Stability Angular Rates/1(alpha beta)
  Mux6/1 -> Stability Angular Rates/2(alphadot betadot)
  1/1 -> Mux6/2
  CG/1 -> Aerodynamic Forces and Moments Stability Axis/3(CG)
  CP/1 -> Aerodynamic Forces and Moments Stability Axis/4(CP)

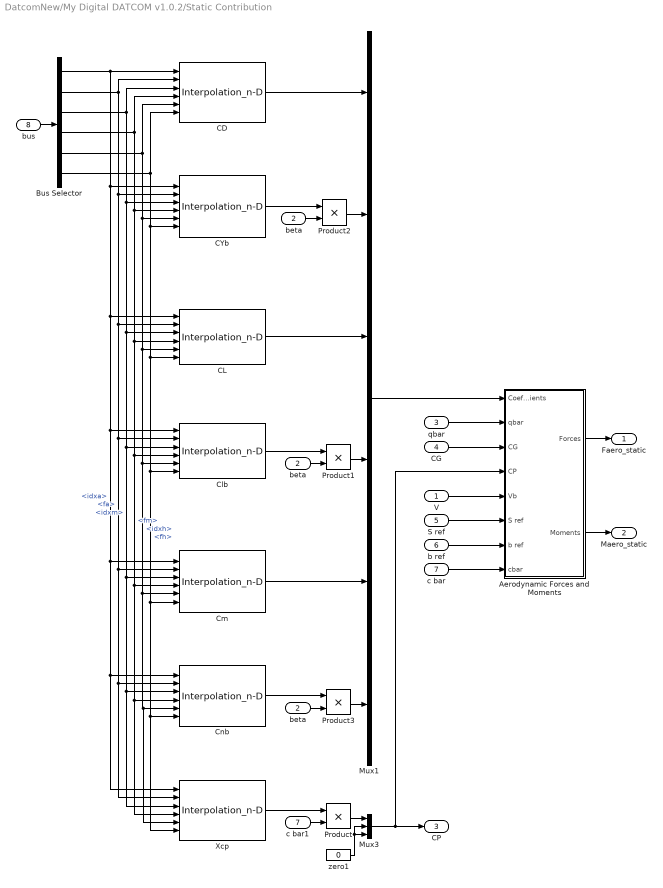
== system DatcomNew/My Digital DATCOM v1.0.2/Static Contribution ==
  "V " : Inport
  beta : Inport  Port=2
  qbar : Inport  Port=3
  CG : Inport  Port=4
  S ref : Inport  Port=5  Unit=m^2
  b ref : Inport  Port=6  Unit=m  PortDimensions=1
  c bar : Inport  Port=7  Unit=m  PortDimensions=1
  bus : Inport  Port=8
  " beta " : InportShadow  Port=2
  Aerodynamic Forces and Moments : Subsystem
  Bus Selector : BusSelector  OutputSignals=idxa,fa,idxm,fm,idxh,fh
  CD : Interpolation_n-D  NumberOfTableDimensions=3  Table=permute(datcom.cd,[1 2 3])  InterpMethod=Flat  ExtrapMethod=Clip  OutDataTypeStr=double
      settings: InputPortMap=u0,u1,u2,u3,u4,u5
  CL : Interpolation_n-D  NumberOfTableDimensions=3  Table=permute(datcom.cl,[1 2 3])  InterpMethod=Flat  ExtrapMethod=Clip  OutDataTypeStr=double
      settings: InputPortMap=u0,u1,u2,u3,u4,u5
  CYb : Interpolation_n-D  NumberOfTableDimensions=3  Table=permute(datcom.cyb,[1 2 3])  InterpMethod=Flat  ExtrapMethod=Clip  OutDataTypeStr=double
      settings: InputPortMap=u0,u1,u2,u3,u4,u5
  Clb : Interpolation_n-D  NumberOfTableDimensions=3  Table=permute(datcom.clb,[1 2 3])  InterpMethod=Flat  ExtrapMethod=Clip  OutDataTypeStr=double
      settings: InputPortMap=u0,u1,u2,u3,u4,u5
  Cm : Interpolation_n-D  NumberOfTableDimensions=3  Table=permute(datcom.cm,[1 2 3])  InterpMethod=Flat  ExtrapMethod=Clip  OutDataTypeStr=double
      settings: InputPortMap=u0,u1,u2,u3,u4,u5
  Cnb : Interpolation_n-D  NumberOfTableDimensions=3  Table=permute(datcom.cnb,[1 2 3])  InterpMethod=Flat  ExtrapMethod=Clip  OutDataTypeStr=double
      settings: InputPortMap=u0,u1,u2,u3,u4,u5
  Mux1 : Mux  Inputs=6
  Mux3 : Mux  Inputs=3
  Product : Product
  Product1 : Product  RndMeth=Zero
  Product2 : Product  RndMeth=Zero
  Product3 : Product  RndMeth=Zero
  Xcp : Interpolation_n-D  NumberOfTableDimensions=3  Table="permute(datcom.xcp,[1  2  3])"  OutDataTypeStr=double
      settings: InputPortMap=u0,u1,u2,u3,u4,u5
  "beta " : InportShadow  Port=2
  c bar1 : InportShadow  Port=7  Unit=m  PortDimensions=1
  zero1 : Constant  Value=0
  Faero_static : Outport
  Maero_static : Outport  Port=2
  "CP " : Outport  Port=3
  wires:
  c bar1/1 -> Product/2
  Product/1 -> Mux3/1
  zero1/1 -> Mux3/3, Mux3/2
  Xcp/1 -> Product/1
  c bar/1 -> Aerodynamic Forces and Moments/8(cbar)
  b ref/1 -> Aerodynamic Forces and Moments/7(b ref)
  S ref/1 -> Aerodynamic Forces and Moments/6(S ref)
  Mux3/1 -> Aerodynamic Forces and Moments/4(CP), "CP "/1
  CG/1 -> Aerodynamic Forces and Moments/3(CG)
  bus/1 -> Bus Selector/1
  Bus Selector/1 -> CD/1, CYb/1, Clb/1, Cnb/1, Xcp/1, Cm/1, CL/1  "<idxa>"
  Bus Selector/2 -> Cnb/2, Xcp/2, Cm/2, Clb/2, CL/2, CYb/2, CD/2  "<fa>"
  Bus Selector/3 -> Cnb/3, Xcp/3, Cm/3, Clb/3, CL/3, CYb/3, CD/3  "<idxm>"
  Bus Selector/4 -> Cnb/4, Xcp/4, Cm/4, Clb/4, CL/4, CYb/4, CD/4  "<fm>"
  Bus Selector/5 -> Cnb/5, Xcp/5, Cm/5, Clb/5, CL/5, CYb/5, CD/5  "<idxh>"
  Bus Selector/6 -> Cnb/6, Xcp/6, Cm/6, Clb/6, CL/6, CYb/6, CD/6  "<fh>"
  CD/1 -> Mux1/1
  CL/1 -> Mux1/3
  CYb/1 -> Product2/1
  beta/1 -> Product2/2
  Clb/1 -> Product1/1
  "beta "/1 -> Product1/2
  Product2/1 -> Mux1/2
  Product1/1 -> Mux1/4
  Cm/1 -> Mux1/5
  Cnb/1 -> Product3/1
  " beta "/1 -> Product3/2
  Product3/1 -> Mux1/6
  Mux1/1 -> Aerodynamic Forces and Moments/1(Coefficients)
  Aerodynamic Forces and Moments/1(Forces) -> Faero_static/1
  qbar/1 -> Aerodynamic Forces and Moments/2(qbar)
  Aerodynamic Forces and Moments/2(Moments) -> Maero_static/1
  "V "/1 -> Aerodynamic Forces and Moments/5(Vb)

== system DatcomNew/My Digital DATCOM v1.0.3/Deflection ==
  CP : Inport
  bus : Inport  Port=2
  "V " : Inport  Port=3
  qbar : Inport  Port=4
  CG : Inport  Port=5
  S ref : Inport  Port=6  Unit=m^2
  b ref : Inport  Port=7  Unit=m  PortDimensions=1
  c bar : Inport  Port=8  Unit=m  PortDimensions=1
  Aerodynamic Forces and Moments : Subsystem
  Delta Coefficients : Subsystem
  delta_Faero : Outport
  delta_Maero : Outport  Port=2
  wires:
  Aerodynamic Forces and Moments/1(Forces) -> delta_Faero/1
  Aerodynamic Forces and Moments/2(Moments) -> delta_Maero/1
  S ref/1 -> Aerodynamic Forces and Moments/6(S ref)
  b ref/1 -> Aerodynamic Forces and Moments/7(b ref)
  qbar/1 -> Aerodynamic Forces and Moments/2(qbar)
  c bar/1 -> Aerodynamic Forces and Moments/8(cbar)
  CG/1 -> Aerodynamic Forces and Moments/3(CG)
  "V "/1 -> Aerodynamic Forces and Moments/5(Vb)
  CP/1 -> Aerodynamic Forces and Moments/4(CP)
  Delta Coefficients/1(delCoeff) -> Aerodynamic Forces and Moments/1(Coefficients)
  bus/1 -> Delta Coefficients/1(bus)

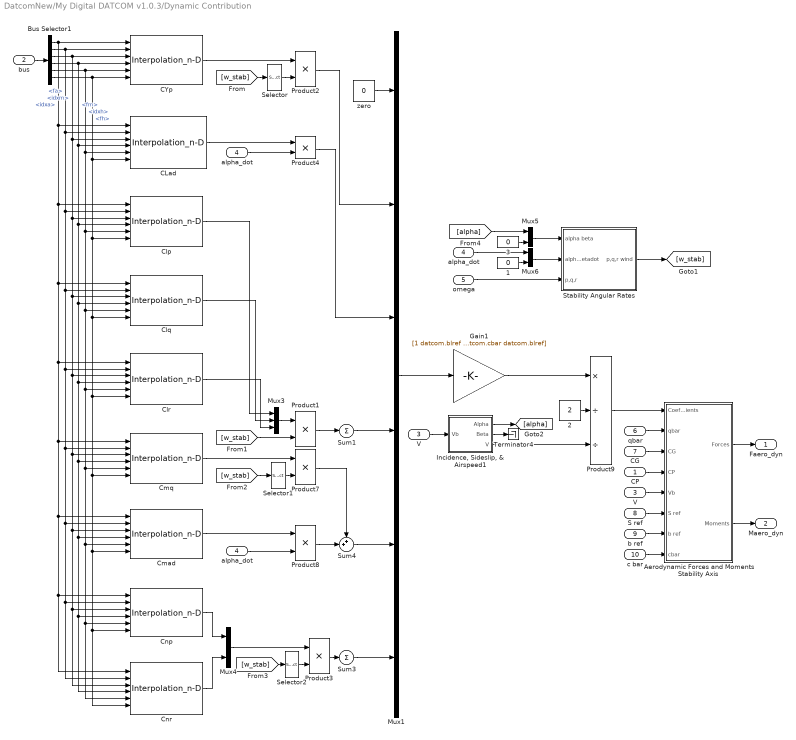
== system DatcomNew/My Digital DATCOM v1.0.3/Dynamic Contribution ==
  CP : Inport
  bus : Inport  Port=2
  V : Inport  Port=3
  alpha_dot : Inport  Port=4  Unit=rad/s
  omega : Inport  Port=5  Unit=rad/s
  qbar : Inport  Port=6
  CG : Inport  Port=7
  S ref : Inport  Port=8  Unit=m^2
  b ref : Inport  Port=9  Unit=m  PortDimensions=1
  c bar : Inport  Port=10  Unit=m  PortDimensions=1
  " V " : InportShadow  Port=3
  " alpha_dot " : InportShadow  Port=4  Unit=rad/s
  1 : Constant  Value=0
  2 : Constant  Value=2
  3 : Constant  Value=0
  Aerodynamic Forces and Moments Stability Axis : Subsystem
  Bus Selector1 : BusSelector  OutputSignals=idxa,fa,idxm,fm,idxh,fh
  CLad : Interpolation_n-D  NumberOfTableDimensions=3  Table="permute(datcom.clad,[1  2  3])"  OutDataTypeStr=double
      settings: InputPortMap=u0,u1,u2,u3,u4,u5
  CYp : Interpolation_n-D  NumberOfTableDimensions=3  Table="permute(datcom.cyp,[1  2  3])"  OutDataTypeStr=double
      settings: InputPortMap=u0,u1,u2,u3,u4,u5
  Clp : Interpolation_n-D  NumberOfTableDimensions=3  Table="permute(datcom.clp,[1  2  3])"  OutDataTypeStr=double
      settings: InputPortMap=u0,u1,u2,u3,u4,u5
  Clq : Interpolation_n-D  NumberOfTableDimensions=3  Table="permute(datcom.clq,[1  2  3])"  OutDataTypeStr=double
      settings: InputPortMap=u0,u1,u2,u3,u4,u5
  Clr : Interpolation_n-D  NumberOfTableDimensions=3  Table="permute(datcom.clr,[1  2  3])"  OutDataTypeStr=double
      settings: InputPortMap=u0,u1,u2,u3,u4,u5
  Cmad : Interpolation_n-D  NumberOfTableDimensions=3  Table="permute(datcom.cmad,[1  2  3])"  OutDataTypeStr=double
      settings: InputPortMap=u0,u1,u2,u3,u4,u5
  Cmq : Interpolation_n-D  NumberOfTableDimensions=3  Table="permute(datcom.cmq,[1  2  3])"  OutDataTypeStr=double
      settings: InputPortMap=u0,u1,u2,u3,u4,u5
  Cnp : Interpolation_n-D  NumberOfTableDimensions=3  Table="permute(datcom.cnp,[1  2  3])"  OutDataTypeStr=double
      settings: InputPortMap=u0,u1,u2,u3,u4,u5
  Cnr : Interpolation_n-D  NumberOfTableDimensions=3  Table="permute(datcom.cnr,[1  2  3])"  OutDataTypeStr=double
      settings: InputPortMap=u0,u1,u2,u3,u4,u5
  Gain1 : Gain  Gain=[1 datcom.blref datcom.cbar datcom.blref datcom.cbar datcom.blref]
  "Incidence, Sideslip, & Airspeed1" : Subsystem
      mask Display:
      | port_label('input',1,'V_b','texmode','on');
      | port_label('output',1,'\alpha','texmode','on');
      | port_label('output',2,'\beta','texmode','on');
      | port_label('output',3,'V','texmode','on');
  Mux1 : Mux  Inputs=6
  Mux3 : Mux  Inputs=3
  Mux4 : Mux  Inputs=2
  Mux5 : Mux  Inputs=2
  Mux6 : Mux  Inputs=2
  Product{1..4,7..8} (6 alike) : Product  RndMeth=Zero
  Product9 : Product  Inputs=*//  RndMeth=Zero
  Selector : Selector  InputPortWidth=3  IndexOptions=Index vector (dialog)  Indices=1  OutputSizes=1
  Selector1 : Selector  InputPortWidth=3  IndexOptions=Index vector (dialog)  Indices=2  OutputSizes=1
  Selector2 : Selector  InputPortWidth=3  IndexOptions=Index vector (dialog)  Indices=[1 3]  OutputSizes=1
  Stability Angular Rates : Subsystem
      mask Display:
      | port_label('input',1,'\alpha \beta','texmode','on');
      | port_label('input',2,'d\alpha/dt d\beta/dt','texmode','on');
      | port_label('input',3,'\omega','texmode','on');
      | port_label('output',1,'\omega_w','texmode','on');
  Sum1 : Sum  Inputs=+
  Sum3 : Sum  Inputs=+
  Sum4 : Sum  Inputs=++|
  Terminator4 : Terminator
  "alpha_dot " : InportShadow  Port=4  Unit=rad/s
  zero : Constant  Value=0
  Faero_dyn : Outport
  Maero_dyn : Outport  Port=2
  wires:
  c bar/1 -> Aerodynamic Forces and Moments Stability Axis/8(cbar)
  b ref/1 -> Aerodynamic Forces and Moments Stability Axis/7(b ref)
  S ref/1 -> Aerodynamic Forces and Moments Stability Axis/6(S ref)
  CLad/1 -> Product4/1
  Bus Selector1/6 -> Clp/6, Clq/6, Clr/6, Cmq/6, Cmad/6, Cnp/6, Cnr/6, CLad/6, CYp/6  "<fh>"
  Bus Selector1/5 -> Clp/5, Clq/5, Clr/5, Cmq/5, Cmad/5, Cnp/5, Cnr/5, CLad/5, CYp/5  "<idxh>"
  Bus Selector1/4 -> Clp/4, Clq/4, Clr/4, Cmq/4, Cmad/4, Cnp/4, Cnr/4, CLad/4, CYp/4  "<fm>"
  Bus Selector1/3 -> Clp/3, Clq/3, Clr/3, Cmq/3, Cmad/3, Cnp/3, Cnr/3, CLad/3, CYp/3  "<idxm>"
  Bus Selector1/2 -> Clp/2, Clq/2, Clr/2, Cmq/2, Cmad/2, Cnp/2, Cnr/2, CLad/2, CYp/2  "<fa>"
  Bus Selector1/1 -> Clp/1, Clq/1, Clr/1, Cmq/1, Cmad/1, Cnp/1, Cnr/1, CLad/1, CYp/1  "<idxa>"
  bus/1 -> Bus Selector1/1
  " alpha_dot "/1 -> Mux6/1
  omega/1 -> Stability Angular Rates/3(p,q,r)
  Stability Angular Rates/1(p,q,r wind) -> [w_stab]
  Mux1/1 -> Gain1/1
  Cnp/1 -> Mux4/1
  Cmq/1 -> Product7/1
  Sum1/1 -> Mux1/4
  Product2/1 -> Mux1/2
  Clq/1 -> Mux3/2
  Selector/1 -> Product2/2
  CYp/1 -> Product2/1
  "alpha_dot "/1 -> Product4/2
  [w_stab] -> Selector/1
  Clr/1 -> Mux3/3
  Clp/1 -> Mux3/1
  Mux3/1 -> Product1/1
  [w_stab] -> Product1/2
  Product1/1 -> Sum1/1
  [w_stab] -> Selector1/1
  Selector1/1 -> Product7/2
  Product7/1 -> Sum4/1
  Cmad/1 -> Product8/1
  Product8/1 -> Sum4/2
  alpha_dot/1 -> Product8/2
  Cnr/1 -> Mux4/2
  [w_stab] -> Selector2/1
  Mux4/1 -> Product3/1
  Selector2/1 -> Product3/2
  Sum3/1 -> Mux1/6
  Product3/1 -> Sum3/1
  Gain1/1 -> Product9/1
  Product9/1 -> Aerodynamic Forces and Moments Stability Axis/1(Coefficients)
  2/1 -> Product9/2
  V/1 -> "Incidence, Sideslip, & Airspeed1"/1(Vb)
  Sum4/1 -> Mux1/5
  Product4/1 -> Mux1/3
  zero/1 -> Mux1/1
  "Incidence, Sideslip, & Airspeed1"/3(V) -> Product9/3
  "Incidence, Sideslip, & Airspeed1"/2(Beta) -> Terminator4/1
  "Incidence, Sideslip, & Airspeed1"/1(Alpha) -> [alpha]
  Aerodynamic Forces and Moments Stability Axis/1(Forces) -> Faero_dyn/1
  qbar/1 -> Aerodynamic Forces and Moments Stability Axis/2(qbar)
  Aerodynamic Forces and Moments Stability Axis/2(Moments) -> Maero_dyn/1
  " V "/1 -> Aerodynamic Forces and Moments Stability Axis/5(Vb)
  3/1 -> Mux5/2
  [alpha] -> Mux5/1
  Mux5/1 -> Stability Angular Rates/1(alpha beta)
  Mux6/1 -> Stability Angular Rates/2(alphadot betadot)
  1/1 -> Mux6/2
  CG/1 -> Aerodynamic Forces and Moments Stability Axis/3(CG)
  CP/1 -> Aerodynamic Forces and Moments Stability Axis/4(CP)
